simulink model "truck_fra_oven"  (R2023b)
settings: Solver=VariableStepAuto  StartTime=0.0  StopTime=80  MaxStep=0.01  RelTol=1e-3
values from neighbouring files (symbols this model uses):
  k_1 = -0.1    [truck_fra_oven_script.m]
  k_2 = 2    [truck_fra_oven_script.m]
  K_i = 10    [truck_fra_oven_script.m]
  K_p = 2000    [truck_fra_oven_script.m]
libraries: simulink x2
settings Model: SimulationMode=accelerator  Creator=hansae  LastModifiedBy=fredr
settings SolverCC: AlgebraicLoopSolver=TrustRegion
settings SFSimCC: CustomCodeUndefinedFunction=UseInterfaceOnly

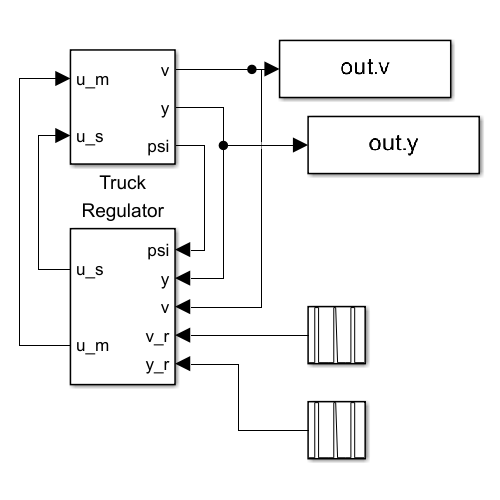
[thumbnail: Simulink's stored preview of the top-level diagram]
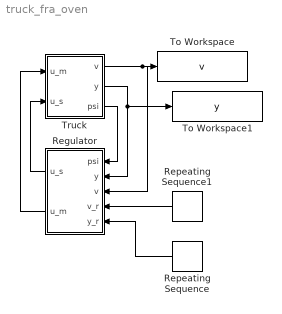
== system truck_fra_oven ==
  Regulator : Subsystem
  Repeating Sequence : simulink/Sources/Repeating Sequence  rep_seq_t=[0 29.9 30 49.9 50 100]  rep_seq_y="[-2 -2 2  2 -2 -2]"
  Repeating Sequence1 : simulink/Sources/Repeating Sequence  rep_seq_t=[0 29.9 30 49.9 50 100]  rep_seq_y=[20 20 30 30 20 20]
  To Workspace : ToWorkspace  VariableName=v  SampleTime=0.1
      settings: Save2DSignal=2-D array (concatenate along first dimension)
  To Workspace1 : ToWorkspace  VariableName=y  SampleTime=0.1
      settings: Save2DSignal=2-D array (concatenate along first dimension)
  Truck : Subsystem
  wires:
  Regulator/2(u_m) -> Truck/1(u_m)
  Regulator/1(u_s) -> Truck/2(u_s)
  Truck/1(v) -> Regulator/3(v), To Workspace/1
  Truck/2(y) -> Regulator/2(y), To Workspace1/1
  Truck/3(psi) -> Regulator/1(psi)
  Repeating Sequence/1 -> Regulator/5(y_r)
  Repeating Sequence1/1 -> Regulator/4(v_r)

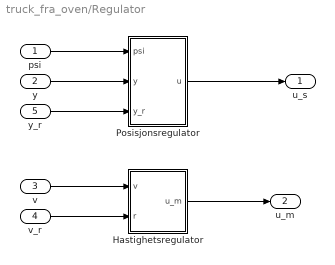
== system truck_fra_oven/Regulator ==
  psi : Inport
  y : Inport  Port=2
  v : Inport  Port=3
  v_r : Inport  Port=4
  y_r : Inport  Port=5
  Hastighetsregulator : Subsystem
  Posisjonsregulator : Subsystem
  u_s : Outport
  u_m : Outport  Port=2
  wires:
  v/1 -> Hastighetsregulator/1(v)
  v_r/1 -> Hastighetsregulator/2(r)
  psi/1 -> Posisjonsregulator/1(psi)
  y_r/1 -> Posisjonsregulator/3(y_r)
  y/1 -> Posisjonsregulator/2(y)
  Hastighetsregulator/1(u_m) -> u_m/1
  Posisjonsregulator/1(u) -> u_s/1

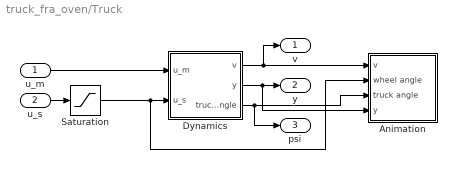
== system truck_fra_oven/Truck ==
  u_m : Inport
  u_s : Inport  Port=2
  Animation : Subsystem
  Dynamics : Subsystem  ClipboardFcn=parameters_truck.m
  Saturation : Saturate  UpperLimit=pi/4  LowerLimit=-pi/4
  v : Outport
  y : Outport  Port=2
  psi : Outport  Port=3
  wires:
  Dynamics/2(y) -> y/1, Animation/4(y)
  u_s/1 -> Saturation/1
  u_m/1 -> Dynamics/1(u_m)
  Dynamics/3(truck angle) -> psi/1, Animation/3(truck angle)
  Saturation/1 -> Animation/2(wheel angle), Dynamics/2(u_s)
  Dynamics/1(v) -> v/1, Animation/1(v)

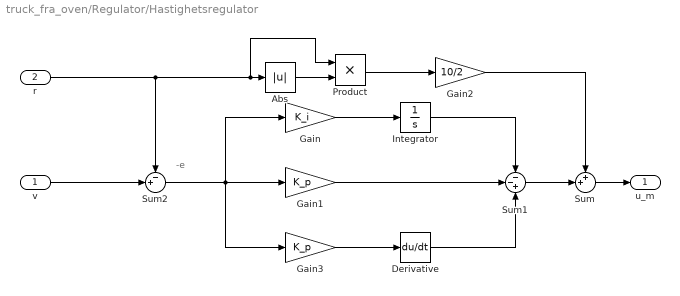
== system truck_fra_oven/Regulator/Hastighetsregulator ==
  note: -e
  v : Inport
  r : Inport  Port=2
  Abs : Abs  SaturateOnIntegerOverflow=off
  Derivative : Derivative
  Gain : Gain  Gain=K_i
  Gain1 : Gain  Gain=K_p
  Gain2 : Gain  Gain=10/2
  Gain3 : Gain  Gain=K_p
  Integrator : Integrator
  Product : Product
  Sum : Sum  Inputs=++|
  Sum1 : Sum  Inputs=--+
  Sum2 : Sum  Inputs=-+|
  u_m : Outport
  wires:
  Sum/1 -> u_m/1
  Gain/1 -> Integrator/1
  Sum1/1 -> Sum/2
  Gain1/1 -> Sum1/2
  Integrator/1 -> Sum1/1
  r/1 -> Product/1, Abs/1, Sum2/1
  Abs/1 -> Product/2
  Product/1 -> Gain2/1
  Gain2/1 -> Sum/1
  v/1 -> Sum2/2
  Sum2/1 -> Gain3/1, Gain1/1, Gain/1
  Gain3/1 -> Derivative/1
  Derivative/1 -> Sum1/3

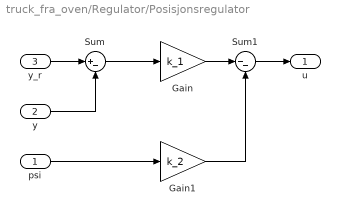
== system truck_fra_oven/Regulator/Posisjonsregulator ==
  psi : Inport
  y : Inport  Port=2
  y_r : Inport  Port=3
  Gain : Gain  Gain=k_1
  Gain1 : Gain  Gain=k_2
  Sum : Sum  Inputs=|+-
  Sum1 : Sum  Inputs=|--
  u : Outport
  wires:
  y_r/1 -> Sum/1
  y/1 -> Sum/2
  Sum/1 -> Gain/1
  psi/1 -> Gain1/1
  Gain/1 -> Sum1/1
  Sum1/1 -> u/1
  Gain1/1 -> Sum1/2

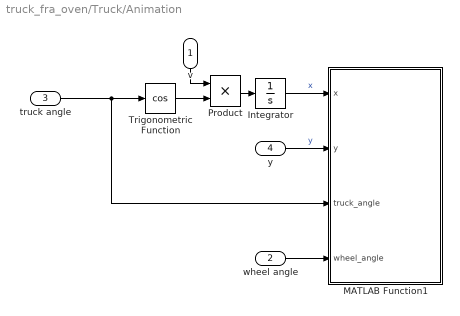
== system truck_fra_oven/Truck/Animation ==
  v : Inport
  wheel angle : Inport  Port=2
  truck angle : Inport  Port=3
  y : Inport  Port=4
  Integrator : Integrator
  MATLAB Function1 : MATLAB Function  TreatAsAtomicUnit=on  SystemSampleTime=1/30
  Product : Product
  Trigonometric Function : Trigonometry  Operator=cos
  wires:
  Product/1 -> Integrator/1
  Trigonometric Function/1 -> Product/2
  v/1 -> Product/1
  y/1 -> MATLAB Function1/2(y)  "y"
  Integrator/1 -> MATLAB Function1/1(x)  "x"
  truck angle/1 -> MATLAB Function1/3(truck_angle), Trigonometric Function/1
  wheel angle/1 -> MATLAB Function1/4(wheel_angle)

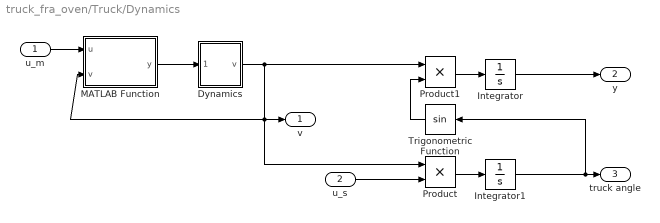
== system truck_fra_oven/Truck/Dynamics ==
  u_m : Inport
  u_s : Inport  Port=2
  Dynamics : Subsystem  ClipboardFcn=parameters_truck.m
  Integrator : Integrator  InitialCondition=-2
  Integrator1 : Integrator
  MATLAB Function : MATLAB Function  TreatAsAtomicUnit=on
  Product : Product
  Product1 : Product
  Trigonometric Function : Trigonometry
  v : Outport
  y : Outport  Port=2
  truck angle : Outport  Port=3
  wires:
  Integrator/1 -> y/1
  Product/1 -> Integrator1/1
  Product1/1 -> Integrator/1
  Trigonometric Function/1 -> Product1/2
  u_s/1 -> Product/2
  Integrator1/1 -> truck angle/1, Trigonometric Function/1
  MATLAB Function/1(y) -> Dynamics/1(u_m)
  u_m/1 -> MATLAB Function/1(u)
  Dynamics/1(v) -> Product/1, MATLAB Function/2(v), v/1, Product1/1

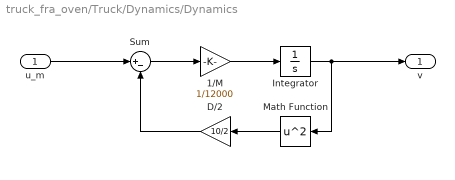
== system truck_fra_oven/Truck/Dynamics/Dynamics ==
  u_m : Inport
  1/M : Gain  Gain=1/12000
  D/2 : Gain  Gain=10/2
  Integrator : Integrator
  Math Function : Math  Operator=square  SignedPower=on
  Sum : Sum  Inputs=|+-
  v : Outport
  wires:
  Integrator/1 -> v/1, Math Function/1
  Sum/1 -> 1/M/1
  u_m/1 -> Sum/1
  1/M/1 -> Integrator/1
  D/2/1 -> Sum/2
  Math Function/1 -> D/2/1

== matlab function truck_fra_oven/Truck/Dynamics/MATLAB Function ==
  data: u input; y output; v input
function y = saturation(u,v)
    Pmax = 400000;
    epsilon = 0.1;
    
    sat = Pmax/sqrt(v^2+epsilon);
    y = max(min(u,sat),-sat);

== matlab function truck_fra_oven/Truck/Animation/MATLAB Function1 ==
  settings: updateMethod=DISCRETE
  data: x input; y input; truck_angle input; wheel_angle input
function plot_truck(x,y,truck_angle,wheel_angle)
    % Parameters
    l = 8;
    persistent Truck;

    % Plotting Truck
    if isempty(Truck)
        Truck = initialize_plot();
    else
        update_truck_position(Truck,x,y,truck_angle,wheel_angle);
    end    

    drawnow;

    % Functions
    function Truck = initialize_plot()
        % Create figure
        figure('position',[100,100,1500,500]);
        clf; grid on; hold on; daspect([1,1,1]);
        xlim([-20, 50])
        ylim([-10, 10])
    
        % Road
        plot([-5000,5000],[-4,-4],'k','linewidth',3);
        plot([-5000,5000],[4,4],'k','linewidth',3);
        plot([-5000,5000],[0,0],'y','linewidth',3);

        % Truck
        Truck               = hgtransform('parent',gca);
        Left_front_wheel    = hgtransform('parent',Truck);
        Right_front_wheel   = hgtransform('parent',Truck);

        % Back wheels
        rectangle('Position',[l/6,-l/100,l/8,l/40],'parent',Truck,'edgecolor','k','linewidth',2,'FaceColor','w')
        rectangle('Position',[l/6,l-2*l/3-(l/40-l/100),l/8,l/40],'parent',Truck,'edgecolor','k','linewidth',2,'FaceColor','w')
        % Front wheel
        rectangle('Position',[2*l/3+l/20,-l/100,l/8,l/40],'parent',Right_front_wheel,'edgecolor','k','linewidth',2,'FaceColor','w')
        rectangle('Position',[2*l/3+l/20,l-2*l/3-(l/40-l/100),l/8,l/40],'parent',Left_front_wheel,'edgecolor','k','linewidth',2,'FaceColor','w')
        % Back
        rectangle('Position',[0,0,11*l/18,l-2*l/3],'parent',Truck,'edgecolor','k','linewidth',2,'FaceColor','w')
        % Front
        rectangle('Position',[2*l/3,0,l-2*l/3,l-2*l/3],'parent',Truck,'edgecolor','k','linewidth',2,'FaceColor','w')
        % Connection
        rectangle('Position',[11*l/18,3*l/8-l/3,2*l/3-11*l/18,l-3*l/4],'parent',Truck,'edgecolor','k','linewidth',2,'FaceColor','w')
        % Window
        rectangle('Position',[7*l/8,0,l/8,l-2*l/3],'parent',Truck,'edgecolor','k','linewidth',2,'FaceColor','w')
        
    end
    
    function update_truck_position(Truck,x,y,truck_angle,wheel_angle)
        if ishandle(Truck)
            set(Truck, 'Matrix', makehgtform('translate', [x, y, 0], 'zrotate', truck_angle, 'translate', [-l/6-l/16, -l/2+l/3, 0]));
            
            children = get(Truck, 'Children');
            set(children(8), 'Matrix', makehgtform('translate', -[-(2*l/3+l/20)-l/16, -(l-2*l/3-(l/40-l/100))-l/80, 0], 'zrotate', -wheel_angle, 'translate', [-(2*l/3+l/20)-l/16, -(l-2*l/3-(l/40-l/100))-l/80, 0]));
            set(children(7), 'Matrix', makehgtform('translate', -[-(2*l/3+l/20)-l/16, l/100-l/80, 0], 'zrotate', -wheel_angle, 'translate', [-(2*l/3+l/20)-l/16, l/100-l/80, 0]));
    
            xlim([-20, 50] + x)
            ylim([-10, 10] + y)
        end
    end
end
